simulink model "pendulum_sim"  (Simulink 8.1)
settings: Solver=ode45  StartTime=0.0  StopTime=60  RelTol=1e-3
settings Model: FrictionCoefficient=0.6  Length=1  initPos=2.3783  initVel=0  Creator=Rudi  LastModifiedBy=rudi
settings DataIOCC: LimitDataPoints=off  SaveFormat=StructureWithTime  SignalLogging=off  ReturnWorkspaceOutputs=on  ReturnWorkspaceOutputsName=sim_out

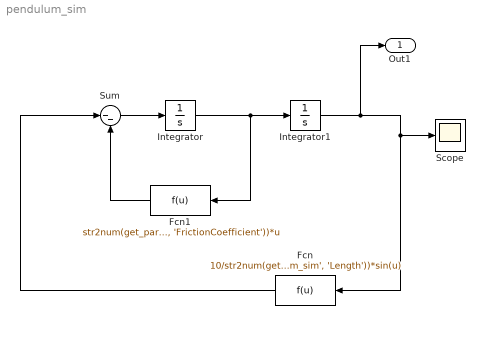
== system pendulum_sim ==
  Fcn : Fcn  Expr=10/str2num(get_param('pendulum_sim', 'Length'))*sin(u)
  Fcn1 : Fcn  Expr=str2num(get_param('pendulum_sim', 'FrictionCoefficient'))*u
  Integrator : Integrator  InitialCondition=str2num(get_param('pendulum_sim', 'initVel'))
  Integrator1 : Integrator  InitialCondition=str2num(get_param('pendulum_sim', 'initPos'))
  Scope : Scope
  Sum : Sum  Inputs=|--
  Out1 : Outport
  wires:
  Integrator/1 -> Integrator1/1, Fcn1/1
  Integrator1/1 -> Out1/1, Fcn/1, Scope/1
  Sum/1 -> Integrator/1
  Fcn/1 -> Sum/1
  Fcn1/1 -> Sum/2
